simulink model "Subsystem"  (R2020b)
settings: Solver=VariableStepAuto  StartTime=0.0  StopTime=10.0  RelTol=1e-3
settings Model: Creator=hp  LastModifiedBy=hp
settings DataIOCC: SaveOutput=off  SaveTime=off

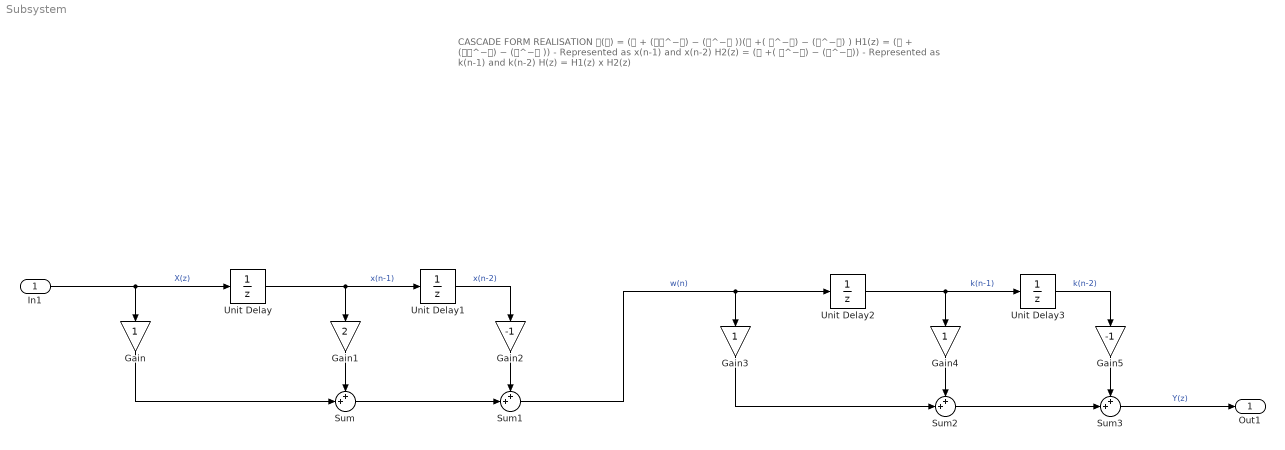
== system Subsystem ==
  note: CASCADE FORM REALISATION
      |
      | 𝐇(𝐳) = (𝟏 + (𝟐𝐳^−𝟏) − (𝐳^−𝟐 ))(𝟏 +( 𝐳^−𝟏) − (𝐳^−𝟐) )
      | H1(z) = (𝟏 + (𝟐𝐳^−𝟏) − (𝐳^−𝟐 )) - Represented as x(n-1) and x(n-2)
      | H2(z) = (𝟏 +( 𝐳^−𝟏) − (𝐳^−𝟐)) - Represented as k(n-1) and k(n-2)
      |
      | H(z) = H1(z) x H2(z)
  In1 : Inport  OutDataTypeStr=double  PortDimensions=1  SampleTime=0
  Gain : Gain
  Gain1 : Gain  Gain=2
  Gain2 : Gain  Gain=-1
  Gain3 : Gain
  Gain4 : Gain
  Gain5 : Gain  Gain=-1
  Sum{,1..3} (4 alike) : Sum  Inputs=++|
  Unit Delay{,1..3} (4 alike) : UnitDelay  SampleTime=-1  HasFrameUpgradeWarning=on
  Out1 : Outport  OutDataTypeStr=double  PortDimensions=1  SampleTime=0
  wires:
  Sum/1 -> Sum1/2
  In1/1 -> Unit Delay/1, Gain/1  "X(z)"
  Gain1/1 -> Sum/1
  Unit Delay/1 -> Unit Delay1/1, Gain1/1  "x(n-1)"
  Unit Delay2/1 -> Unit Delay3/1, Gain4/1  "k(n-1)"
  Unit Delay1/1 -> Gain2/1  "x(n-2)"
  Gain4/1 -> Sum2/1
  Gain2/1 -> Sum1/1
  Sum1/1 -> Unit Delay2/1, Gain3/1  "w(n)"
  Unit Delay3/1 -> Gain5/1  "k(n-2)"
  Gain5/1 -> Sum3/1
  Sum2/1 -> Sum3/2
  Gain3/1 -> Sum2/2
  Gain/1 -> Sum/2
  Sum3/1 -> Out1/1  "Y(z)"
